simulink model "Ultrafiltration"  (R2025b)
settings: Solver=FixedStepAuto  StartTime=0.0  StopTime=1440  FixedStep=1  RelTol=1e-3
InitFcn:
  | initUF
  | tic;
StartFcn:
  | disp("Start...")
StopFcn:
  | disp("Stop...")
  | fprintf("SimTime: %.02f min", toc/60)
values from neighbouring files (symbols this model uses):
  BW_Max_Time = 90    [initUF.m]
  BW_Max_Vol_gal = 5000    [initUF.m]
  CEB_Max_Time = 1000    [initUF.m]
  CEB_Max_Vol_gal = 5000    [initUF.m]
  CIP_Max_Time = 15000    [initUF.m]
undefined symbols (not defined in the file or in its folder): LUT
libraries: simulink x30
(part 3 of 5)

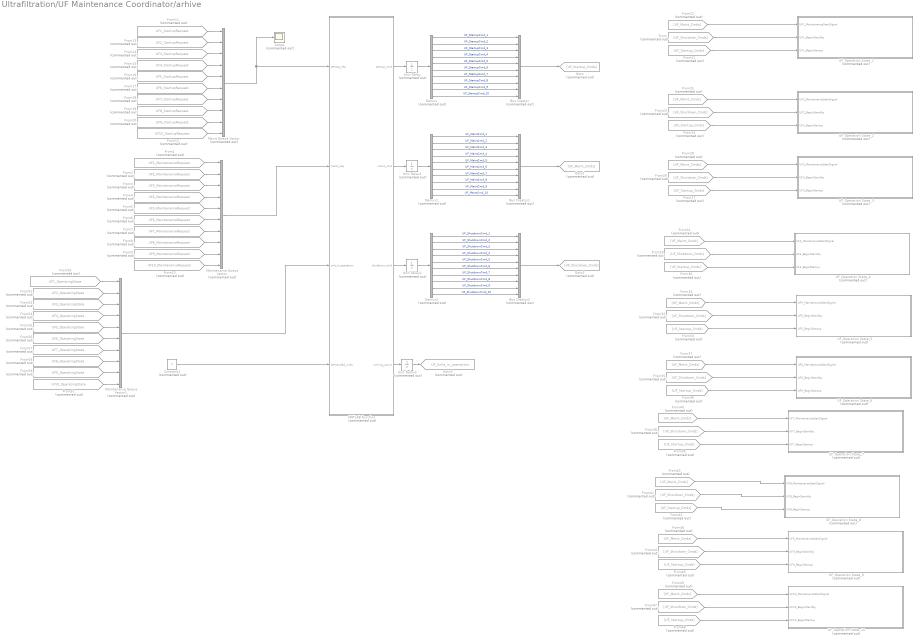
== system Ultrafiltration/UF Maintenance Coordinator/arhive ==
  Bus Creator : BusCreator  Commented=on  Inputs=10
  Bus Creator1 : BusCreator  Commented=on  Inputs=10
  Bus Creator2 : BusCreator  Commented=on  Inputs=10
  Constant1 : Constant  Commented=on  Value=7
  Demux : Demux  Commented=on  Outputs=10
  Demux1 : Demux  Commented=on  Outputs=10
  Demux2 : Demux  Commented=on  Outputs=10
  From{,23,26,29,32,35,38,41,44,47} (10 alike) : From  Commented=on  GotoTag=UF_Shutdown_Cmds
  From1 : From  Commented=on  GotoTag=UF1_MaintenanceRequest  TagVisibility=global
  From10 : From  Commented=on  GotoTag=UF10_MaintenanceRequest  TagVisibility=global
  From11 : From  Commented=on  GotoTag=UF1_StartupRequest  TagVisibility=global
  From12 : From  Commented=on  GotoTag=UF10_StartupRequest  TagVisibility=global
  From13 : From  Commented=on  GotoTag=UF2_StartupRequest  TagVisibility=global
  From14 : From  Commented=on  GotoTag=UF3_StartupRequest  TagVisibility=global
  From15 : From  Commented=on  GotoTag=UF4_StartupRequest  TagVisibility=global
  From16 : From  Commented=on  GotoTag=UF5_StartupRequest  TagVisibility=global
  From17 : From  Commented=on  GotoTag=UF6_StartupRequest  TagVisibility=global
  From18 : From  Commented=on  GotoTag=UF7_StartupRequest  TagVisibility=global
  From19 : From  Commented=on  GotoTag=UF8_StartupRequest  TagVisibility=global
  From2 : From  Commented=on  GotoTag=UF2_MaintenanceRequest  TagVisibility=global
  From20 : From  Commented=on  GotoTag=UF9_StartupRequest  TagVisibility=global
  From{21,24,27,30,33,36,39,42,45,48} (10 alike) : From  Commented=on  GotoTag=UF_Startup_Cmds
  From{22,25,28,31,34,37,40,43,46,49} (10 alike) : From  Commented=on  GotoTag=UF_Maint_Cmds
  From3 : From  Commented=on  GotoTag=UF3_MaintenanceRequest  TagVisibility=global
  From4 : From  Commented=on  GotoTag=UF4_MaintenanceRequest  TagVisibility=global
  From5 : From  Commented=on  GotoTag=UF5_MaintenanceRequest  TagVisibility=global
  From50 : From  Commented=on  GotoTag=UF1_OperatingState  TagVisibility=global
  From51 : From  Commented=on  GotoTag=UF10_OperatingState  TagVisibility=global
  From52 : From  Commented=on  GotoTag=UF2_OperatingState  TagVisibility=global
  From53 : From  Commented=on  GotoTag=UF3_OperatingState  TagVisibility=global
  From54 : From  Commented=on  GotoTag=UF4_OperatingState  TagVisibility=global
  From55 : From  Commented=on  GotoTag=UF5_OperatingState  TagVisibility=global
  From56 : From  Commented=on  GotoTag=UF6_OperatingState  TagVisibility=global
  From57 : From  Commented=on  GotoTag=UF7_OperatingState  TagVisibility=global
  From58 : From  Commented=on  GotoTag=UF8_OperatingState  TagVisibility=global
  From59 : From  Commented=on  GotoTag=UF9_OperatingState  TagVisibility=global
  From6 : From  Commented=on  GotoTag=UF6_MaintenanceRequest  TagVisibility=global
  From7 : From  Commented=on  GotoTag=UF7_MaintenanceRequest  TagVisibility=global
  From8 : From  Commented=on  GotoTag=UF8_MaintenanceRequest  TagVisibility=global
  From9 : From  Commented=on  GotoTag=UF9_MaintenanceRequest  TagVisibility=global
  Goto : Goto  Commented=on  GotoTag=UF_Startup_Cmds
  Goto1 : Goto  Commented=on  GotoTag=UF_Maint_Cmds
  Goto2 : Goto  Commented=on  GotoTag=UF_Shutdown_Cmds
  Goto3 : Goto  Commented=on  GotoTag=UF_Units_in_operations  TagVisibility=global
  MATLAB Function : MATLAB Function  Priority=100  Commented=on  TreatAsAtomicUnit=on
  Maint Queue Vector : Mux  Commented=on  Inputs=10
  Maintenance Queue Vector : Mux  Commented=on  Inputs=10
  Maintenance Queue Vector1 : Mux  Commented=on  Inputs=10
  Scope : Scope  Commented=on
      settings: ActiveDisplayYMinimum=0.31827009128781919  ActiveDisplayYMaximum=0.91954146390153213
  UF_Operation State_1 : Subsystem  Commented=on
  UF_Operation State_10 : Subsystem  Commented=on
  UF_Operation State_2 : Subsystem  Commented=on
  UF_Operation State_3 : Subsystem  Commented=on
  UF_Operation State_4 : Subsystem  Commented=on
  UF_Operation State_5 : Subsystem  Commented=on
  UF_Operation State_6 : Subsystem  Commented=on
  UF_Operation State_7 : Subsystem  Commented=on
  UF_Operation State_8 : Subsystem  Commented=on
  UF_Operation State_9 : Subsystem  Commented=on
  Unit Delay{,1..3} (4 alike) : UnitDelay  Commented=on  SampleTime=-1  HasFrameUpgradeWarning=on
  wires:
  Demux2/9 -> Bus Creator2/9  "UF_ShutdownCmd_9"
  From13/1 -> Maint Queue Vector/2
  From42/1 -> UF_Operation State_8/3(UF8_BeginStartup)
  From48/1 -> UF_Operation State_10/3(UF10_BeginStartup)
  Demux2/10 -> Bus Creator2/10  "UF_ShutdownCmd_10"
  From47/1 -> UF_Operation State_10/2(UF10_BeginStandby)
  Demux2/6 -> Bus Creator2/6  "UF_ShutdownCmd_6"
  Demux1/6 -> Bus Creator1/6  "UF_MaintCmd_6"
  From24/1 -> UF_Operation State_2/3(UF2_BeginStartup)
  Maintenance Queue Vector/1 -> MATLAB Function/2(maint_req)
  From1/1 -> Maintenance Queue Vector/1
  From23/1 -> UF_Operation State_2/2(UF2_BeginStandby)
  MATLAB Function/3(shutdown_cmd) -> Unit Delay2/1
  From30/1 -> UF_Operation State_4/3(UF4_BeginStartup)
  From57/1 -> Maintenance Queue Vector1/7
  Unit Delay/1 -> Demux/1
  Demux/10 -> Bus Creator/10  "UF_StartupCmd_10"
  From54/1 -> Maintenance Queue Vector1/4
  From45/1 -> UF_Operation State_9/3(UF9_BeginStartup)
  Demux1/2 -> Bus Creator1/2  "UF_MaintCmd_2"
  From7/1 -> Maintenance Queue Vector/7
  From58/1 -> Maintenance Queue Vector1/8
  From49/1 -> UF_Operation State_10/1(UF10_MaintenanceStartSignal)
  From29/1 -> UF_Operation State_4/2(UF4_BeginStandby)
  From6/1 -> Maintenance Queue Vector/6
  From10/1 -> Maintenance Queue Vector/10
  From56/1 -> Maintenance Queue Vector1/6
  From33/1 -> UF_Operation State_5/3(UF5_BeginStartup)
  From31/1 -> UF_Operation State_4/1(UF4_MaintenanceStartSignal)
  From/1 -> UF_Operation State_1/2(UF1_BeginStandby)
  From53/1 -> Maintenance Queue Vector1/3
  From34/1 -> UF_Operation State_5/1(UF5_MaintenanceStartSignal)
  Demux2/5 -> Bus Creator2/5  "UF_ShutdownCmd_5"
  Unit Delay3/1 -> Goto3/1
  From59/1 -> Maintenance Queue Vector1/9
  Demux/7 -> Bus Creator/7  "UF_StartupCmd_7"
  Maintenance Queue Vector1/1 -> MATLAB Function/3(unit_in_operation)
  Demux2/7 -> Bus Creator2/7  "UF_ShutdownCmd_7"
  From3/1 -> Maintenance Queue Vector/3
  From38/1 -> UF_Operation State_7/2(UF7_BeginStandby)
  From40/1 -> UF_Operation State_7/1(UF7_MaintenanceStartSignal)
  From26/1 -> UF_Operation State_3/2(UF3_BeginStandby)
  Bus Creator1/1 -> Goto1/1
  From2/1 -> Maintenance Queue Vector/2
  Demux2/3 -> Bus Creator2/3  "UF_ShutdownCmd_3"
  From39/1 -> UF_Operation State_7/3(UF7_BeginStartup)
  Demux1/9 -> Bus Creator1/9  "UF_MaintCmd_9"
  Demux2/2 -> Bus Creator2/2  "UF_ShutdownCmd_2"
  From46/1 -> UF_Operation State_9/1(UF9_MaintenanceStartSignal)
  From20/1 -> Maint Queue Vector/9
  Demux/4 -> Bus Creator/4  "UF_StartupCmd_4"
  Demux2/4 -> Bus Creator2/4  "UF_ShutdownCmd_4"
  Demux/5 -> Bus Creator/5  "UF_StartupCmd_5"
  Demux2/1 -> Bus Creator2/1  "UF_ShutdownCmd_1"
  From9/1 -> Maintenance Queue Vector/9
  From32/1 -> UF_Operation State_5/2(UF5_BeginStandby)
  Demux1/3 -> Bus Creator1/3  "UF_MaintCmd_3"
  Demux1/5 -> Bus Creator1/5  "UF_MaintCmd_5"
  From55/1 -> Maintenance Queue Vector1/5
  From4/1 -> Maintenance Queue Vector/4
  MATLAB Function/4(running_count) -> Unit Delay3/1
  Demux/6 -> Bus Creator/6  "UF_StartupCmd_6"
  From22/1 -> UF_Operation State_1/1(UF1_MaintenanceStartSignal)
  Demux/8 -> Bus Creator/8  "UF_StartupCmd_8"
  Demux/9 -> Bus Creator/9  "UF_StartupCmd_9"
  From8/1 -> Maintenance Queue Vector/8
  Demux1/1 -> Bus Creator1/1  "UF_MaintCmd_1"
  Demux1/10 -> Bus Creator1/10  "UF_MaintCmd_10"
  From50/1 -> Maintenance Queue Vector1/1
  Demux1/4 -> Bus Creator1/4  "UF_MaintCmd_4"
  MATLAB Function/1(startup_cmd) -> Unit Delay/1
  From52/1 -> Maintenance Queue Vector1/2
  From27/1 -> UF_Operation State_3/3(UF3_BeginStartup)
  From15/1 -> Maint Queue Vector/4
  From51/1 -> Maintenance Queue Vector1/10
  From36/1 -> UF_Operation State_6/3(UF6_BeginStartup)
  MATLAB Function/2(maint_cmd) -> Unit Delay1/1
  Unit Delay2/1 -> Demux2/1
  From43/1 -> UF_Operation State_8/1(UF8_MaintenanceStartSignal)
  From28/1 -> UF_Operation State_3/1(UF3_MaintenanceStartSignal)
  Demux2/8 -> Bus Creator2/8  "UF_ShutdownCmd_8"
  Demux/2 -> Bus Creator/2  "UF_StartupCmd_2"
  From35/1 -> UF_Operation State_6/2(UF6_BeginStandby)
  Bus Creator2/1 -> Goto2/1
  Bus Creator/1 -> Goto/1
  From37/1 -> UF_Operation State_6/1(UF6_MaintenanceStartSignal)
  Constant1/1 -> MATLAB Function/4(demanded_units)
  Demux1/8 -> Bus Creator1/8  "UF_MaintCmd_8"
  From25/1 -> UF_Operation State_2/1(UF2_MaintenanceStartSignal)
  From44/1 -> UF_Operation State_9/2(UF9_BeginStandby)
  Demux1/7 -> Bus Creator1/7  "UF_MaintCmd_7"
  Demux/3 -> Bus Creator/3  "UF_StartupCmd_3"
  Demux/1 -> Bus Creator/1  "UF_StartupCmd_1"
  From41/1 -> UF_Operation State_8/2(UF8_BeginStandby)
  From21/1 -> UF_Operation State_1/3(UF1_BeginStartup)
  From5/1 -> Maintenance Queue Vector/5
  Unit Delay1/1 -> Demux1/1
  From16/1 -> Maint Queue Vector/5
  From17/1 -> Maint Queue Vector/6
  From19/1 -> Maint Queue Vector/8
  From11/1 -> Maint Queue Vector/1
  From12/1 -> Maint Queue Vector/10
  From18/1 -> Maint Queue Vector/7
  Maint Queue Vector/1 -> Scope/1, MATLAB Function/1(startup_req)
  From14/1 -> Maint Queue Vector/3

== system Ultrafiltration/UF1/Subsystem ==
  note: The GAM utilizes smoothing functions to generate non-interacting linear regressions between the parameters. The format of the equation is as such:
      | $y = \beta_0 + \sum_{n=1}^N{f_n(x_n)}\\ f_n(x_n) = \beta_{n}*sm_n(x_n)$
      | where f_n is the weighted smoothing function for variable n across the set N. Each 1-D lookup table below represents the weighted smooth function output for the respective variable. This GAM lookup table approach provided a more computationally efficient method to predict using the GAM at very minor losses in fidelity ( ~0.1% MAPE from raw GAM outputs across a test set).
  t_BW : Inport
  t_CEB : Inport  Port=2
  t_CIP : Inport  Port=3
  V_BW : Inport  Port=4
  V_CEB : Inport  Port=5
  Feed Turbidity : Inport  Port=6
  T : Inport  Port=7
  B1: t_BW : Lookup_n-D  NumberOfTableDimensions=1  BreakpointsForDimension1=LUT.breakpoints(:,3)  Table=LUT.values(:,3)  ExtrapMethod=Clip  InternalRulePriority=Speed  RndMeth=Simplest
  B2: t_CEB : Lookup_n-D  NumberOfTableDimensions=1  BreakpointsForDimension1=LUT.breakpoints(:,5)  Table=LUT.values(:,5)  ExtrapMethod=Clip  InternalRulePriority=Speed  RndMeth=Simplest
  B3: t_CIP : Lookup_n-D  NumberOfTableDimensions=1  BreakpointsForDimension1=LUT.breakpoints(:,4)  Table=LUT.values(:,4)  ExtrapMethod=Clip  InternalRulePriority=Speed  RndMeth=Simplest
  B4: V_BW : Lookup_n-D  NumberOfTableDimensions=1  BreakpointsForDimension1=LUT.breakpoints(:,6)  Table=LUT.values(:,6)  ExtrapMethod=Clip  InternalRulePriority=Speed  RndMeth=Simplest
  B5: V_CEB : Lookup_n-D  NumberOfTableDimensions=1  BreakpointsForDimension1=LUT.breakpoints(:,7)  Table=LUT.values(:,7)  ExtrapMethod=Clip  InternalRulePriority=Speed  RndMeth=Simplest
  B6: Turbidity : Lookup_n-D  NumberOfTableDimensions=1  BreakpointsForDimension1=LUT.breakpoints(:,1)  Table=LUT.values(:,1)  ExtrapMethod=Clip  InternalRulePriority=Speed  RndMeth=Simplest
  B7: Temperature : Lookup_n-D  NumberOfTableDimensions=1  BreakpointsForDimension1=LUT.breakpoints(:,2)  Table=LUT.values(:,2)  ExtrapMethod=Clip  InternalRulePriority=Speed  RndMeth=Simplest
  Intercept : Constant  Value=LUT.intercept
  Sum : Sum  Inputs=++++++++
  A_UF : Outport
  wires:
  Sum/1 -> A_UF/1
  t_BW/1 -> B1: t_BW/1
  B1: t_BW/1 -> Sum/2
  Intercept/1 -> Sum/1
  t_CEB/1 -> B2: t_CEB/1
  B2: t_CEB/1 -> Sum/3
  t_CIP/1 -> B3: t_CIP/1
  B3: t_CIP/1 -> Sum/4
  V_BW/1 -> B4: V_BW/1
  B4: V_BW/1 -> Sum/5
  V_CEB/1 -> B5: V_CEB/1
  B5: V_CEB/1 -> Sum/6
  B6: Turbidity/1 -> Sum/7
  Feed Turbidity/1 -> B6: Turbidity/1
  T/1 -> B7: Temperature/1
  B7: Temperature/1 -> Sum/8

== system Ultrafiltration/UF10/Subsystem ==
  note: The GAM utilizes smoothing functions to generate non-interacting linear regressions between the parameters. The format of the equation is as such:
      | $y = \beta_0 + \sum_{n=1}^N{f_n(x_n)}\\ f_n(x_n) = \beta_{n}*sm_n(x_n)$
      | where f_n is the weighted smoothing function for variable n across the set N. Each 1-D lookup table below represents the weighted smooth function output for the respective variable. This GAM lookup table approach provided a more computationally efficient method to predict using the GAM at very minor losses in fidelity ( ~0.1% MAPE from raw GAM outputs across a test set).
  t_BW : Inport
  t_CEB : Inport  Port=2
  t_CIP : Inport  Port=3
  V_BW : Inport  Port=4
  V_CEB : Inport  Port=5
  Feed Turbidity : Inport  Port=6
  T : Inport  Port=7
  B1: t_BW : Lookup_n-D  NumberOfTableDimensions=1  BreakpointsForDimension1=LUT.breakpoints(:,3)  Table=LUT.values(:,3)  ExtrapMethod=Clip  InternalRulePriority=Speed  RndMeth=Simplest
  B2: t_CEB : Lookup_n-D  NumberOfTableDimensions=1  BreakpointsForDimension1=LUT.breakpoints(:,5)  Table=LUT.values(:,5)  ExtrapMethod=Clip  InternalRulePriority=Speed  RndMeth=Simplest
  B3: t_CIP : Lookup_n-D  NumberOfTableDimensions=1  BreakpointsForDimension1=LUT.breakpoints(:,4)  Table=LUT.values(:,4)  ExtrapMethod=Clip  InternalRulePriority=Speed  RndMeth=Simplest
  B4: V_BW : Lookup_n-D  NumberOfTableDimensions=1  BreakpointsForDimension1=LUT.breakpoints(:,6)  Table=LUT.values(:,6)  ExtrapMethod=Clip  InternalRulePriority=Speed  RndMeth=Simplest
  B5: V_CEB : Lookup_n-D  NumberOfTableDimensions=1  BreakpointsForDimension1=LUT.breakpoints(:,7)  Table=LUT.values(:,7)  ExtrapMethod=Clip  InternalRulePriority=Speed  RndMeth=Simplest
  B6: Turbidity : Lookup_n-D  NumberOfTableDimensions=1  BreakpointsForDimension1=LUT.breakpoints(:,1)  Table=LUT.values(:,1)  ExtrapMethod=Clip  InternalRulePriority=Speed  RndMeth=Simplest
  B7: Temperature : Lookup_n-D  NumberOfTableDimensions=1  BreakpointsForDimension1=LUT.breakpoints(:,2)  Table=LUT.values(:,2)  ExtrapMethod=Clip  InternalRulePriority=Speed  RndMeth=Simplest
  Intercept : Constant  Value=LUT.intercept
  Sum : Sum  Inputs=++++++++
  A_UF : Outport
  wires:
  Sum/1 -> A_UF/1
  t_BW/1 -> B1: t_BW/1
  B1: t_BW/1 -> Sum/2
  Intercept/1 -> Sum/1
  t_CEB/1 -> B2: t_CEB/1
  B2: t_CEB/1 -> Sum/3
  t_CIP/1 -> B3: t_CIP/1
  B3: t_CIP/1 -> Sum/4
  V_BW/1 -> B4: V_BW/1
  B4: V_BW/1 -> Sum/5
  V_CEB/1 -> B5: V_CEB/1
  B5: V_CEB/1 -> Sum/6
  B6: Turbidity/1 -> Sum/7
  Feed Turbidity/1 -> B6: Turbidity/1
  T/1 -> B7: Temperature/1
  B7: Temperature/1 -> Sum/8

== system Ultrafiltration/UF2/Subsystem ==
  note: The GAM utilizes smoothing functions to generate non-interacting linear regressions between the parameters. The format of the equation is as such:
      | $y = \beta_0 + \sum_{n=1}^N{f_n(x_n)}\\ f_n(x_n) = \beta_{n}*sm_n(x_n)$
      | where f_n is the weighted smoothing function for variable n across the set N. Each 1-D lookup table below represents the weighted smooth function output for the respective variable. This GAM lookup table approach provided a more computationally efficient method to predict using the GAM at very minor losses in fidelity ( ~0.1% MAPE from raw GAM outputs across a test set).
  t_BW : Inport
  t_CEB : Inport  Port=2
  t_CIP : Inport  Port=3
  V_BW : Inport  Port=4
  V_CEB : Inport  Port=5
  Feed Turbidity : Inport  Port=6
  T : Inport  Port=7
  B1: t_BW : Lookup_n-D  NumberOfTableDimensions=1  BreakpointsForDimension1=LUT.breakpoints(:,3)  Table=LUT.values(:,3)  ExtrapMethod=Clip  InternalRulePriority=Speed  RndMeth=Simplest
  B2: t_CEB : Lookup_n-D  NumberOfTableDimensions=1  BreakpointsForDimension1=LUT.breakpoints(:,5)  Table=LUT.values(:,5)  ExtrapMethod=Clip  InternalRulePriority=Speed  RndMeth=Simplest
  B3: t_CIP : Lookup_n-D  NumberOfTableDimensions=1  BreakpointsForDimension1=LUT.breakpoints(:,4)  Table=LUT.values(:,4)  ExtrapMethod=Clip  InternalRulePriority=Speed  RndMeth=Simplest
  B4: V_BW : Lookup_n-D  NumberOfTableDimensions=1  BreakpointsForDimension1=LUT.breakpoints(:,6)  Table=LUT.values(:,6)  ExtrapMethod=Clip  InternalRulePriority=Speed  RndMeth=Simplest
  B5: V_CEB : Lookup_n-D  NumberOfTableDimensions=1  BreakpointsForDimension1=LUT.breakpoints(:,7)  Table=LUT.values(:,7)  ExtrapMethod=Clip  InternalRulePriority=Speed  RndMeth=Simplest
  B6: Turbidity : Lookup_n-D  NumberOfTableDimensions=1  BreakpointsForDimension1=LUT.breakpoints(:,1)  Table=LUT.values(:,1)  ExtrapMethod=Clip  InternalRulePriority=Speed  RndMeth=Simplest
  B7: Temperature : Lookup_n-D  NumberOfTableDimensions=1  BreakpointsForDimension1=LUT.breakpoints(:,2)  Table=LUT.values(:,2)  ExtrapMethod=Clip  InternalRulePriority=Speed  RndMeth=Simplest
  Intercept : Constant  Value=LUT.intercept
  Sum : Sum  Inputs=++++++++
  A_UF : Outport
  wires:
  Sum/1 -> A_UF/1
  t_BW/1 -> B1: t_BW/1
  B1: t_BW/1 -> Sum/2
  Intercept/1 -> Sum/1
  t_CEB/1 -> B2: t_CEB/1
  B2: t_CEB/1 -> Sum/3
  t_CIP/1 -> B3: t_CIP/1
  B3: t_CIP/1 -> Sum/4
  V_BW/1 -> B4: V_BW/1
  B4: V_BW/1 -> Sum/5
  V_CEB/1 -> B5: V_CEB/1
  B5: V_CEB/1 -> Sum/6
  B6: Turbidity/1 -> Sum/7
  Feed Turbidity/1 -> B6: Turbidity/1
  T/1 -> B7: Temperature/1
  B7: Temperature/1 -> Sum/8

== system Ultrafiltration/UF3/Subsystem ==
  note: The GAM utilizes smoothing functions to generate non-interacting linear regressions between the parameters. The format of the equation is as such:
      | $y = \beta_0 + \sum_{n=1}^N{f_n(x_n)}\\ f_n(x_n) = \beta_{n}*sm_n(x_n)$
      | where f_n is the weighted smoothing function for variable n across the set N. Each 1-D lookup table below represents the weighted smooth function output for the respective variable. This GAM lookup table approach provided a more computationally efficient method to predict using the GAM at very minor losses in fidelity ( ~0.1% MAPE from raw GAM outputs across a test set).
  t_BW : Inport
  t_CEB : Inport  Port=2
  t_CIP : Inport  Port=3
  V_BW : Inport  Port=4
  V_CEB : Inport  Port=5
  Feed Turbidity : Inport  Port=6
  T : Inport  Port=7
  B1: t_BW : Lookup_n-D  NumberOfTableDimensions=1  BreakpointsForDimension1=LUT.breakpoints(:,3)  Table=LUT.values(:,3)  ExtrapMethod=Clip  InternalRulePriority=Speed  RndMeth=Simplest
  B2: t_CEB : Lookup_n-D  NumberOfTableDimensions=1  BreakpointsForDimension1=LUT.breakpoints(:,5)  Table=LUT.values(:,5)  ExtrapMethod=Clip  InternalRulePriority=Speed  RndMeth=Simplest
  B3: t_CIP : Lookup_n-D  NumberOfTableDimensions=1  BreakpointsForDimension1=LUT.breakpoints(:,4)  Table=LUT.values(:,4)  ExtrapMethod=Clip  InternalRulePriority=Speed  RndMeth=Simplest
  B4: V_BW : Lookup_n-D  NumberOfTableDimensions=1  BreakpointsForDimension1=LUT.breakpoints(:,6)  Table=LUT.values(:,6)  ExtrapMethod=Clip  InternalRulePriority=Speed  RndMeth=Simplest
  B5: V_CEB : Lookup_n-D  NumberOfTableDimensions=1  BreakpointsForDimension1=LUT.breakpoints(:,7)  Table=LUT.values(:,7)  ExtrapMethod=Clip  InternalRulePriority=Speed  RndMeth=Simplest
  B6: Turbidity : Lookup_n-D  NumberOfTableDimensions=1  BreakpointsForDimension1=LUT.breakpoints(:,1)  Table=LUT.values(:,1)  ExtrapMethod=Clip  InternalRulePriority=Speed  RndMeth=Simplest
  B7: Temperature : Lookup_n-D  NumberOfTableDimensions=1  BreakpointsForDimension1=LUT.breakpoints(:,2)  Table=LUT.values(:,2)  ExtrapMethod=Clip  InternalRulePriority=Speed  RndMeth=Simplest
  Intercept : Constant  Value=LUT.intercept
  Sum : Sum  Inputs=++++++++
  A_UF : Outport
  wires:
  Sum/1 -> A_UF/1
  t_BW/1 -> B1: t_BW/1
  B1: t_BW/1 -> Sum/2
  Intercept/1 -> Sum/1
  t_CEB/1 -> B2: t_CEB/1
  B2: t_CEB/1 -> Sum/3
  t_CIP/1 -> B3: t_CIP/1
  B3: t_CIP/1 -> Sum/4
  V_BW/1 -> B4: V_BW/1
  B4: V_BW/1 -> Sum/5
  V_CEB/1 -> B5: V_CEB/1
  B5: V_CEB/1 -> Sum/6
  B6: Turbidity/1 -> Sum/7
  Feed Turbidity/1 -> B6: Turbidity/1
  T/1 -> B7: Temperature/1
  B7: Temperature/1 -> Sum/8

== system Ultrafiltration/UF4/Subsystem ==
  note: The GAM utilizes smoothing functions to generate non-interacting linear regressions between the parameters. The format of the equation is as such:
      | $y = \beta_0 + \sum_{n=1}^N{f_n(x_n)}\\ f_n(x_n) = \beta_{n}*sm_n(x_n)$
      | where f_n is the weighted smoothing function for variable n across the set N. Each 1-D lookup table below represents the weighted smooth function output for the respective variable. This GAM lookup table approach provided a more computationally efficient method to predict using the GAM at very minor losses in fidelity ( ~0.1% MAPE from raw GAM outputs across a test set).
  t_BW : Inport
  t_CEB : Inport  Port=2
  t_CIP : Inport  Port=3
  V_BW : Inport  Port=4
  V_CEB : Inport  Port=5
  Feed Turbidity : Inport  Port=6
  T : Inport  Port=7
  B1: t_BW : Lookup_n-D  NumberOfTableDimensions=1  BreakpointsForDimension1=LUT.breakpoints(:,3)  Table=LUT.values(:,3)  ExtrapMethod=Clip  InternalRulePriority=Speed  RndMeth=Simplest
  B2: t_CEB : Lookup_n-D  NumberOfTableDimensions=1  BreakpointsForDimension1=LUT.breakpoints(:,5)  Table=LUT.values(:,5)  ExtrapMethod=Clip  InternalRulePriority=Speed  RndMeth=Simplest
  B3: t_CIP : Lookup_n-D  NumberOfTableDimensions=1  BreakpointsForDimension1=LUT.breakpoints(:,4)  Table=LUT.values(:,4)  ExtrapMethod=Clip  InternalRulePriority=Speed  RndMeth=Simplest
  B4: V_BW : Lookup_n-D  NumberOfTableDimensions=1  BreakpointsForDimension1=LUT.breakpoints(:,6)  Table=LUT.values(:,6)  ExtrapMethod=Clip  InternalRulePriority=Speed  RndMeth=Simplest
  B5: V_CEB : Lookup_n-D  NumberOfTableDimensions=1  BreakpointsForDimension1=LUT.breakpoints(:,7)  Table=LUT.values(:,7)  ExtrapMethod=Clip  InternalRulePriority=Speed  RndMeth=Simplest
  B6: Turbidity : Lookup_n-D  NumberOfTableDimensions=1  BreakpointsForDimension1=LUT.breakpoints(:,1)  Table=LUT.values(:,1)  ExtrapMethod=Clip  InternalRulePriority=Speed  RndMeth=Simplest
  B7: Temperature : Lookup_n-D  NumberOfTableDimensions=1  BreakpointsForDimension1=LUT.breakpoints(:,2)  Table=LUT.values(:,2)  ExtrapMethod=Clip  InternalRulePriority=Speed  RndMeth=Simplest
  Intercept : Constant  Value=LUT.intercept
  Sum : Sum  Inputs=++++++++
  A_UF : Outport
  wires:
  Sum/1 -> A_UF/1
  t_BW/1 -> B1: t_BW/1
  B1: t_BW/1 -> Sum/2
  Intercept/1 -> Sum/1
  t_CEB/1 -> B2: t_CEB/1
  B2: t_CEB/1 -> Sum/3
  t_CIP/1 -> B3: t_CIP/1
  B3: t_CIP/1 -> Sum/4
  V_BW/1 -> B4: V_BW/1
  B4: V_BW/1 -> Sum/5
  V_CEB/1 -> B5: V_CEB/1
  B5: V_CEB/1 -> Sum/6
  B6: Turbidity/1 -> Sum/7
  Feed Turbidity/1 -> B6: Turbidity/1
  T/1 -> B7: Temperature/1
  B7: Temperature/1 -> Sum/8

== system Ultrafiltration/UF5/Subsystem ==
  note: The GAM utilizes smoothing functions to generate non-interacting linear regressions between the parameters. The format of the equation is as such:
      | $y = \beta_0 + \sum_{n=1}^N{f_n(x_n)}\\ f_n(x_n) = \beta_{n}*sm_n(x_n)$
      | where f_n is the weighted smoothing function for variable n across the set N. Each 1-D lookup table below represents the weighted smooth function output for the respective variable. This GAM lookup table approach provided a more computationally efficient method to predict using the GAM at very minor losses in fidelity ( ~0.1% MAPE from raw GAM outputs across a test set).
  t_BW : Inport
  t_CEB : Inport  Port=2
  t_CIP : Inport  Port=3
  V_BW : Inport  Port=4
  V_CEB : Inport  Port=5
  Feed Turbidity : Inport  Port=6
  T : Inport  Port=7
  B1: t_BW : Lookup_n-D  NumberOfTableDimensions=1  BreakpointsForDimension1=LUT.breakpoints(:,3)  Table=LUT.values(:,3)  ExtrapMethod=Clip  InternalRulePriority=Speed  RndMeth=Simplest
  B2: t_CEB : Lookup_n-D  NumberOfTableDimensions=1  BreakpointsForDimension1=LUT.breakpoints(:,5)  Table=LUT.values(:,5)  ExtrapMethod=Clip  InternalRulePriority=Speed  RndMeth=Simplest
  B3: t_CIP : Lookup_n-D  NumberOfTableDimensions=1  BreakpointsForDimension1=LUT.breakpoints(:,4)  Table=LUT.values(:,4)  ExtrapMethod=Clip  InternalRulePriority=Speed  RndMeth=Simplest
  B4: V_BW : Lookup_n-D  NumberOfTableDimensions=1  BreakpointsForDimension1=LUT.breakpoints(:,6)  Table=LUT.values(:,6)  ExtrapMethod=Clip  InternalRulePriority=Speed  RndMeth=Simplest
  B5: V_CEB : Lookup_n-D  NumberOfTableDimensions=1  BreakpointsForDimension1=LUT.breakpoints(:,7)  Table=LUT.values(:,7)  ExtrapMethod=Clip  InternalRulePriority=Speed  RndMeth=Simplest
  B6: Turbidity : Lookup_n-D  NumberOfTableDimensions=1  BreakpointsForDimension1=LUT.breakpoints(:,1)  Table=LUT.values(:,1)  ExtrapMethod=Clip  InternalRulePriority=Speed  RndMeth=Simplest
  B7: Temperature : Lookup_n-D  NumberOfTableDimensions=1  BreakpointsForDimension1=LUT.breakpoints(:,2)  Table=LUT.values(:,2)  ExtrapMethod=Clip  InternalRulePriority=Speed  RndMeth=Simplest
  Intercept : Constant  Value=LUT.intercept
  Sum : Sum  Inputs=++++++++
  A_UF : Outport
  wires:
  Sum/1 -> A_UF/1
  t_BW/1 -> B1: t_BW/1
  B1: t_BW/1 -> Sum/2
  Intercept/1 -> Sum/1
  t_CEB/1 -> B2: t_CEB/1
  B2: t_CEB/1 -> Sum/3
  t_CIP/1 -> B3: t_CIP/1
  B3: t_CIP/1 -> Sum/4
  V_BW/1 -> B4: V_BW/1
  B4: V_BW/1 -> Sum/5
  V_CEB/1 -> B5: V_CEB/1
  B5: V_CEB/1 -> Sum/6
  B6: Turbidity/1 -> Sum/7
  Feed Turbidity/1 -> B6: Turbidity/1
  T/1 -> B7: Temperature/1
  B7: Temperature/1 -> Sum/8

== system Ultrafiltration/UF6/Subsystem ==
  note: The GAM utilizes smoothing functions to generate non-interacting linear regressions between the parameters. The format of the equation is as such:
      | $y = \beta_0 + \sum_{n=1}^N{f_n(x_n)}\\ f_n(x_n) = \beta_{n}*sm_n(x_n)$
      | where f_n is the weighted smoothing function for variable n across the set N. Each 1-D lookup table below represents the weighted smooth function output for the respective variable. This GAM lookup table approach provided a more computationally efficient method to predict using the GAM at very minor losses in fidelity ( ~0.1% MAPE from raw GAM outputs across a test set).
  t_BW : Inport
  t_CEB : Inport  Port=2
  t_CIP : Inport  Port=3
  V_BW : Inport  Port=4
  V_CEB : Inport  Port=5
  Feed Turbidity : Inport  Port=6
  T : Inport  Port=7
  B1: t_BW : Lookup_n-D  NumberOfTableDimensions=1  BreakpointsForDimension1=LUT.breakpoints(:,3)  Table=LUT.values(:,3)  ExtrapMethod=Clip  InternalRulePriority=Speed  RndMeth=Simplest
  B2: t_CEB : Lookup_n-D  NumberOfTableDimensions=1  BreakpointsForDimension1=LUT.breakpoints(:,5)  Table=LUT.values(:,5)  ExtrapMethod=Clip  InternalRulePriority=Speed  RndMeth=Simplest
  B3: t_CIP : Lookup_n-D  NumberOfTableDimensions=1  BreakpointsForDimension1=LUT.breakpoints(:,4)  Table=LUT.values(:,4)  ExtrapMethod=Clip  InternalRulePriority=Speed  RndMeth=Simplest
  B4: V_BW : Lookup_n-D  NumberOfTableDimensions=1  BreakpointsForDimension1=LUT.breakpoints(:,6)  Table=LUT.values(:,6)  ExtrapMethod=Clip  InternalRulePriority=Speed  RndMeth=Simplest
  B5: V_CEB : Lookup_n-D  NumberOfTableDimensions=1  BreakpointsForDimension1=LUT.breakpoints(:,7)  Table=LUT.values(:,7)  ExtrapMethod=Clip  InternalRulePriority=Speed  RndMeth=Simplest
  B6: Turbidity : Lookup_n-D  NumberOfTableDimensions=1  BreakpointsForDimension1=LUT.breakpoints(:,1)  Table=LUT.values(:,1)  ExtrapMethod=Clip  InternalRulePriority=Speed  RndMeth=Simplest
  B7: Temperature : Lookup_n-D  NumberOfTableDimensions=1  BreakpointsForDimension1=LUT.breakpoints(:,2)  Table=LUT.values(:,2)  ExtrapMethod=Clip  InternalRulePriority=Speed  RndMeth=Simplest
  Intercept : Constant  Value=LUT.intercept
  Sum : Sum  Inputs=++++++++
  A_UF : Outport
  wires:
  Sum/1 -> A_UF/1
  t_BW/1 -> B1: t_BW/1
  B1: t_BW/1 -> Sum/2
  Intercept/1 -> Sum/1
  t_CEB/1 -> B2: t_CEB/1
  B2: t_CEB/1 -> Sum/3
  t_CIP/1 -> B3: t_CIP/1
  B3: t_CIP/1 -> Sum/4
  V_BW/1 -> B4: V_BW/1
  B4: V_BW/1 -> Sum/5
  V_CEB/1 -> B5: V_CEB/1
  B5: V_CEB/1 -> Sum/6
  B6: Turbidity/1 -> Sum/7
  Feed Turbidity/1 -> B6: Turbidity/1
  T/1 -> B7: Temperature/1
  B7: Temperature/1 -> Sum/8

== system Ultrafiltration/UF7/Subsystem ==
  note: The GAM utilizes smoothing functions to generate non-interacting linear regressions between the parameters. The format of the equation is as such:
      | $y = \beta_0 + \sum_{n=1}^N{f_n(x_n)}\\ f_n(x_n) = \beta_{n}*sm_n(x_n)$
      | where f_n is the weighted smoothing function for variable n across the set N. Each 1-D lookup table below represents the weighted smooth function output for the respective variable. This GAM lookup table approach provided a more computationally efficient method to predict using the GAM at very minor losses in fidelity ( ~0.1% MAPE from raw GAM outputs across a test set).
  t_BW : Inport
  t_CEB : Inport  Port=2
  t_CIP : Inport  Port=3
  V_BW : Inport  Port=4
  V_CEB : Inport  Port=5
  Feed Turbidity : Inport  Port=6
  T : Inport  Port=7
  B1: t_BW : Lookup_n-D  NumberOfTableDimensions=1  BreakpointsForDimension1=LUT.breakpoints(:,3)  Table=LUT.values(:,3)  ExtrapMethod=Clip  InternalRulePriority=Speed  RndMeth=Simplest
  B2: t_CEB : Lookup_n-D  NumberOfTableDimensions=1  BreakpointsForDimension1=LUT.breakpoints(:,5)  Table=LUT.values(:,5)  ExtrapMethod=Clip  InternalRulePriority=Speed  RndMeth=Simplest
  B3: t_CIP : Lookup_n-D  NumberOfTableDimensions=1  BreakpointsForDimension1=LUT.breakpoints(:,4)  Table=LUT.values(:,4)  ExtrapMethod=Clip  InternalRulePriority=Speed  RndMeth=Simplest
  B4: V_BW : Lookup_n-D  NumberOfTableDimensions=1  BreakpointsForDimension1=LUT.breakpoints(:,6)  Table=LUT.values(:,6)  ExtrapMethod=Clip  InternalRulePriority=Speed  RndMeth=Simplest
  B5: V_CEB : Lookup_n-D  NumberOfTableDimensions=1  BreakpointsForDimension1=LUT.breakpoints(:,7)  Table=LUT.values(:,7)  ExtrapMethod=Clip  InternalRulePriority=Speed  RndMeth=Simplest
  B6: Turbidity : Lookup_n-D  NumberOfTableDimensions=1  BreakpointsForDimension1=LUT.breakpoints(:,1)  Table=LUT.values(:,1)  ExtrapMethod=Clip  InternalRulePriority=Speed  RndMeth=Simplest
  B7: Temperature : Lookup_n-D  NumberOfTableDimensions=1  BreakpointsForDimension1=LUT.breakpoints(:,2)  Table=LUT.values(:,2)  ExtrapMethod=Clip  InternalRulePriority=Speed  RndMeth=Simplest
  Intercept : Constant  Value=LUT.intercept
  Sum : Sum  Inputs=++++++++
  A_UF : Outport
  wires:
  Sum/1 -> A_UF/1
  t_BW/1 -> B1: t_BW/1
  B1: t_BW/1 -> Sum/2
  Intercept/1 -> Sum/1
  t_CEB/1 -> B2: t_CEB/1
  B2: t_CEB/1 -> Sum/3
  t_CIP/1 -> B3: t_CIP/1
  B3: t_CIP/1 -> Sum/4
  V_BW/1 -> B4: V_BW/1
  B4: V_BW/1 -> Sum/5
  V_CEB/1 -> B5: V_CEB/1
  B5: V_CEB/1 -> Sum/6
  B6: Turbidity/1 -> Sum/7
  Feed Turbidity/1 -> B6: Turbidity/1
  T/1 -> B7: Temperature/1
  B7: Temperature/1 -> Sum/8

== system Ultrafiltration/UF8/Subsystem ==
  note: The GAM utilizes smoothing functions to generate non-interacting linear regressions between the parameters. The format of the equation is as such:
      | $y = \beta_0 + \sum_{n=1}^N{f_n(x_n)}\\ f_n(x_n) = \beta_{n}*sm_n(x_n)$
      | where f_n is the weighted smoothing function for variable n across the set N. Each 1-D lookup table below represents the weighted smooth function output for the respective variable. This GAM lookup table approach provided a more computationally efficient method to predict using the GAM at very minor losses in fidelity ( ~0.1% MAPE from raw GAM outputs across a test set).
  t_BW : Inport
  t_CEB : Inport  Port=2
  t_CIP : Inport  Port=3
  V_BW : Inport  Port=4
  V_CEB : Inport  Port=5
  Feed Turbidity : Inport  Port=6
  T : Inport  Port=7
  B1: t_BW : Lookup_n-D  NumberOfTableDimensions=1  BreakpointsForDimension1=LUT.breakpoints(:,3)  Table=LUT.values(:,3)  ExtrapMethod=Clip  InternalRulePriority=Speed  RndMeth=Simplest
  B2: t_CEB : Lookup_n-D  NumberOfTableDimensions=1  BreakpointsForDimension1=LUT.breakpoints(:,5)  Table=LUT.values(:,5)  ExtrapMethod=Clip  InternalRulePriority=Speed  RndMeth=Simplest
  B3: t_CIP : Lookup_n-D  NumberOfTableDimensions=1  BreakpointsForDimension1=LUT.breakpoints(:,4)  Table=LUT.values(:,4)  ExtrapMethod=Clip  InternalRulePriority=Speed  RndMeth=Simplest
  B4: V_BW : Lookup_n-D  NumberOfTableDimensions=1  BreakpointsForDimension1=LUT.breakpoints(:,6)  Table=LUT.values(:,6)  ExtrapMethod=Clip  InternalRulePriority=Speed  RndMeth=Simplest
  B5: V_CEB : Lookup_n-D  NumberOfTableDimensions=1  BreakpointsForDimension1=LUT.breakpoints(:,7)  Table=LUT.values(:,7)  ExtrapMethod=Clip  InternalRulePriority=Speed  RndMeth=Simplest
  B6: Turbidity : Lookup_n-D  NumberOfTableDimensions=1  BreakpointsForDimension1=LUT.breakpoints(:,1)  Table=LUT.values(:,1)  ExtrapMethod=Clip  InternalRulePriority=Speed  RndMeth=Simplest
  B7: Temperature : Lookup_n-D  NumberOfTableDimensions=1  BreakpointsForDimension1=LUT.breakpoints(:,2)  Table=LUT.values(:,2)  ExtrapMethod=Clip  InternalRulePriority=Speed  RndMeth=Simplest
  Intercept : Constant  Value=LUT.intercept
  Sum : Sum  Inputs=++++++++
  A_UF : Outport
  wires:
  Sum/1 -> A_UF/1
  t_BW/1 -> B1: t_BW/1
  B1: t_BW/1 -> Sum/2
  Intercept/1 -> Sum/1
  t_CEB/1 -> B2: t_CEB/1
  B2: t_CEB/1 -> Sum/3
  t_CIP/1 -> B3: t_CIP/1
  B3: t_CIP/1 -> Sum/4
  V_BW/1 -> B4: V_BW/1
  B4: V_BW/1 -> Sum/5
  V_CEB/1 -> B5: V_CEB/1
  B5: V_CEB/1 -> Sum/6
  B6: Turbidity/1 -> Sum/7
  Feed Turbidity/1 -> B6: Turbidity/1
  T/1 -> B7: Temperature/1
  B7: Temperature/1 -> Sum/8

== system Ultrafiltration/UF9/Subsystem ==
  note: The GAM utilizes smoothing functions to generate non-interacting linear regressions between the parameters. The format of the equation is as such:
      | $y = \beta_0 + \sum_{n=1}^N{f_n(x_n)}\\ f_n(x_n) = \beta_{n}*sm_n(x_n)$
      | where f_n is the weighted smoothing function for variable n across the set N. Each 1-D lookup table below represents the weighted smooth function output for the respective variable. This GAM lookup table approach provided a more computationally efficient method to predict using the GAM at very minor losses in fidelity ( ~0.1% MAPE from raw GAM outputs across a test set).
  t_BW : Inport
  t_CEB : Inport  Port=2
  t_CIP : Inport  Port=3
  V_BW : Inport  Port=4
  V_CEB : Inport  Port=5
  Feed Turbidity : Inport  Port=6
  T : Inport  Port=7
  B1: t_BW : Lookup_n-D  NumberOfTableDimensions=1  BreakpointsForDimension1=LUT.breakpoints(:,3)  Table=LUT.values(:,3)  ExtrapMethod=Clip  InternalRulePriority=Speed  RndMeth=Simplest
  B2: t_CEB : Lookup_n-D  NumberOfTableDimensions=1  BreakpointsForDimension1=LUT.breakpoints(:,5)  Table=LUT.values(:,5)  ExtrapMethod=Clip  InternalRulePriority=Speed  RndMeth=Simplest
  B3: t_CIP : Lookup_n-D  NumberOfTableDimensions=1  BreakpointsForDimension1=LUT.breakpoints(:,4)  Table=LUT.values(:,4)  ExtrapMethod=Clip  InternalRulePriority=Speed  RndMeth=Simplest
  B4: V_BW : Lookup_n-D  NumberOfTableDimensions=1  BreakpointsForDimension1=LUT.breakpoints(:,6)  Table=LUT.values(:,6)  ExtrapMethod=Clip  InternalRulePriority=Speed  RndMeth=Simplest
  B5: V_CEB : Lookup_n-D  NumberOfTableDimensions=1  BreakpointsForDimension1=LUT.breakpoints(:,7)  Table=LUT.values(:,7)  ExtrapMethod=Clip  InternalRulePriority=Speed  RndMeth=Simplest
  B6: Turbidity : Lookup_n-D  NumberOfTableDimensions=1  BreakpointsForDimension1=LUT.breakpoints(:,1)  Table=LUT.values(:,1)  ExtrapMethod=Clip  InternalRulePriority=Speed  RndMeth=Simplest
  B7: Temperature : Lookup_n-D  NumberOfTableDimensions=1  BreakpointsForDimension1=LUT.breakpoints(:,2)  Table=LUT.values(:,2)  ExtrapMethod=Clip  InternalRulePriority=Speed  RndMeth=Simplest
  Intercept : Constant  Value=LUT.intercept
  Sum : Sum  Inputs=++++++++
  A_UF : Outport
  wires:
  Sum/1 -> A_UF/1
  t_BW/1 -> B1: t_BW/1
  B1: t_BW/1 -> Sum/2
  Intercept/1 -> Sum/1
  t_CEB/1 -> B2: t_CEB/1
  B2: t_CEB/1 -> Sum/3
  t_CIP/1 -> B3: t_CIP/1
  B3: t_CIP/1 -> Sum/4
  V_BW/1 -> B4: V_BW/1
  B4: V_BW/1 -> Sum/5
  V_CEB/1 -> B5: V_CEB/1
  B5: V_CEB/1 -> Sum/6
  B6: Turbidity/1 -> Sum/7
  Feed Turbidity/1 -> B6: Turbidity/1
  T/1 -> B7: Temperature/1
  B7: Temperature/1 -> Sum/8

== system Ultrafiltration/UF Maintenance Coordinator/arhive/UF_Operation State_1 ==
  UF1_MaintenanceStartSignal : Inport
  UF1_BeginStandby : Inport  Port=2
  UF1_BeginStartup : Inport  Port=3
  Bus Creator : BusCreator  Inputs=2
  Bus Selector : BusSelector  OutputSignals=UF_ShutdownCmd_1
  Bus Selector1 : BusSelector  OutputSignals=UF_MaintCmd_1
  Bus Selector2 : BusSelector  OutputSignals=UF_StartupCmd_1
  Delay Reset Signal : Memory
  Delay Startup : Memory
  UF1_Maintenance State : Stateflow chart  TreatAsAtomicUnit=on
  tag scope: UF1_MaintenanceRequest=global, UF1_MaintenanceState=global, UF1_OperatingState=global, UF1_StartupRequest=global
  wires:
  UF1_Maintenance State/1(unit_in_maint_queue) -> [UF1_MaintenanceRequest]  "UF1_MaintenanceRequestQueue"
  Bus Creator/1 -> [UF1_MaintenanceState]
  Delay Startup/1 -> [UF1_OperatingState], Bus Creator/1  "UF1_OperationsState"
  UF1_Maintenance State/4(maintenance_completion_indicator) -> Delay Reset Signal/1  "UF1_MaintenanceCompletionSignal"
  [UF1_Maintenance_Request] -> UF1_Maintenance State/2(maint_req)
  Delay Reset Signal/1 -> Bus Creator/2  "UF1_MaintenanceCompletionSignal"
  UF1_Maintenance State/3(unit_in_operation) -> Delay Startup/1  "UF1_OperationsState"
  UF1_Maintenance State/2(unit_in_startup_queue) -> [UF1_StartupRequest]  "UF1_StartupRequestQueue"
  UF1_BeginStandby/1 -> Bus Selector/1  "UF1_BeginStandby"
  Bus Selector/1 -> UF1_Maintenance State/3(standby_cmd)  "<UF_ShutdownCmd_1>"
  UF1_MaintenanceStartSignal/1 -> Bus Selector1/1  "UF1_MaintenanceStartSignal"
  Bus Selector1/1 -> UF1_Maintenance State/1(maint_cmd)  "<UF_MaintCmd_1>"
  UF1_BeginStartup/1 -> Bus Selector2/1  "UF1_BeginStartup"
  Bus Selector2/1 -> UF1_Maintenance State/4(startup_cmd)  "<UF_StartupCmd_1>"

== system Ultrafiltration/UF Maintenance Coordinator/arhive/UF_Operation State_10 ==
  UF10_MaintenanceStartSignal : Inport
  UF10_BeginStandby : Inport  Port=2
  UF10_BeginStartup : Inport  Port=3
  Bus Creator : BusCreator  Inputs=2
  Bus Selector : BusSelector  OutputSignals=UF_ShutdownCmd_10
  Bus Selector10 : BusSelector  OutputSignals=UF_MaintCmd_10
  Bus Selector2 : BusSelector  OutputSignals=UF_StartupCmd_10
  Delay Reset Signal : Memory
  Delay Startup : Memory
  UF10_Maintenance State : Stateflow chart  TreatAsAtomicUnit=on
  tag scope: UF10_MaintenanceRequest=global, UF10_MaintenanceState=global, UF10_OperatingState=global, UF10_StartupRequest=global
  wires:
  UF10_Maintenance State/1(unit_in_maint_queue) -> [UF10_MaintenanceRequest]  "UF10_MaintenanceRequestQueue"
  Bus Creator/1 -> [UF10_MaintenanceState]
  Delay Startup/1 -> [UF10_OperatingState], Bus Creator/1  "UF10_OperationsState"
  UF10_Maintenance State/4(maintenance_completion_indicator) -> Delay Reset Signal/1  "UF10_MaintenanceCompletionSignal"
  [UF10_Maintenance_Request] -> UF10_Maintenance State/2(maint_req)
  Delay Reset Signal/1 -> Bus Creator/2  "UF10_MaintenanceCompletionSignal"
  UF10_Maintenance State/3(unit_in_operation) -> Delay Startup/1  "UF10_OperationsState"
  UF10_Maintenance State/2(unit_in_startup_queue) -> [UF10_StartupRequest]  "UF10_StartupRequestQueue"
  UF10_BeginStandby/1 -> Bus Selector/1  "UF10_BeginStandby"
  Bus Selector/1 -> UF10_Maintenance State/3(standby_cmd)  "<UF_ShutdownCmd_10>"
  UF10_MaintenanceStartSignal/1 -> Bus Selector10/1  "UF10_MaintenanceStartSignal"
  Bus Selector10/1 -> UF10_Maintenance State/1(maint_cmd)  "<UF_MaintCmd_10>"
  UF10_BeginStartup/1 -> Bus Selector2/1  "UF10_BeginStartup"
  Bus Selector2/1 -> UF10_Maintenance State/4(startup_cmd)  "<UF_StartupCmd_10>"

== system Ultrafiltration/UF Maintenance Coordinator/arhive/UF_Operation State_2 ==
  UF2_MaintenanceStartSignal : Inport
  UF2_BeginStandby : Inport  Port=2
  UF2_BeginStartup : Inport  Port=3
  Bus Creator : BusCreator  Inputs=2
  Bus Selector : BusSelector  OutputSignals=UF_ShutdownCmd_2
  Bus Selector1 : BusSelector  OutputSignals=UF_MaintCmd_2
  Bus Selector2 : BusSelector  OutputSignals=UF_StartupCmd_2
  Delay Reset Signal : Memory
  Delay Startup : Memory
  UF2_Maintenance State : Stateflow chart  TreatAsAtomicUnit=on
  tag scope: UF2_MaintenanceRequest=global, UF2_MaintenanceState=global, UF2_OperatingState=global, UF2_StartupRequest=global
  wires:
  UF2_Maintenance State/1(unit_in_maint_queue) -> [UF2_MaintenanceRequest]  "UF2_MaintenanceRequestQueue"
  Bus Creator/1 -> [UF2_MaintenanceState]
  UF2_Maintenance State/4(maintenance_completion_indicator) -> Delay Reset Signal/1  "UF2_MaintenanceCompletionSignal"
  [UF2_Maintenance_Request] -> UF2_Maintenance State/2(maint_req)
  Delay Reset Signal/1 -> Bus Creator/2  "UF2_MaintenanceCompletionSignal"
  UF2_Maintenance State/3(unit_in_operation) -> Delay Startup/1  "UF2_OperationsState"
  UF2_Maintenance State/2(unit_in_startup_queue) -> [UF2_StartupRequest]  "UF2_StartupRequestQueue"
  UF2_BeginStandby/1 -> Bus Selector/1  "UF2_BeginStandby"
  Bus Selector/1 -> UF2_Maintenance State/3(standby_cmd)  "<UF_ShutdownCmd_2>"
  UF2_MaintenanceStartSignal/1 -> Bus Selector1/1  "UF2_MaintenanceStartSignal"
  Bus Selector1/1 -> UF2_Maintenance State/1(maint_cmd)  "<UF_MaintCmd_2>"
  UF2_BeginStartup/1 -> Bus Selector2/1  "UF2_BeginStartup"
  Bus Selector2/1 -> UF2_Maintenance State/4(startup_cmd)  "<UF_StartupCmd_2>"
  Delay Startup/1 -> [UF2_OperatingState], Bus Creator/1  "UF2_OperationsState"

== system Ultrafiltration/UF Maintenance Coordinator/arhive/UF_Operation State_3 ==
  UF3_MaintenanceStartSignal : Inport
  UF3_BeginStandby : Inport  Port=2
  UF3_BeginStartup : Inport  Port=3
  Bus Creator : BusCreator  Inputs=2
  Bus Selector : BusSelector  OutputSignals=UF_ShutdownCmd_3
  Bus Selector2 : BusSelector  OutputSignals=UF_StartupCmd_3
  Bus Selector3 : BusSelector  OutputSignals=UF_MaintCmd_3
  Delay Reset Signal : Memory
  Delay Startup : Memory
  UF3_Maintenance State : Stateflow chart  TreatAsAtomicUnit=on
  tag scope: UF3_MaintenanceRequest=global, UF3_MaintenanceState=global, UF3_OperatingState=global, UF3_StartupRequest=global
  wires:
  UF3_Maintenance State/1(unit_in_maint_queue) -> [UF3_MaintenanceRequest]  "UF3_MaintenanceRequestQueue"
  Bus Creator/1 -> [UF3_MaintenanceState]
  Delay Startup/1 -> [UF3_OperatingState], Bus Creator/1  "UF3_OperationsState"
  UF3_Maintenance State/4(maintenance_completion_indicator) -> Delay Reset Signal/1  "UF3_MaintenanceCompletionSignal"
  [UF3_Maintenance_Request] -> UF3_Maintenance State/2(maint_req)
  Delay Reset Signal/1 -> Bus Creator/2  "UF3_MaintenanceCompletionSignal"
  UF3_Maintenance State/3(unit_in_operation) -> Delay Startup/1  "UF3_OperationsState"
  UF3_Maintenance State/2(unit_in_startup_queue) -> [UF3_StartupRequest]  "UF3_StartupRequestQueue"
  UF3_BeginStandby/1 -> Bus Selector/1  "UF3_BeginStandby"
  Bus Selector/1 -> UF3_Maintenance State/3(standby_cmd)  "<UF_ShutdownCmd_3>"
  UF3_MaintenanceStartSignal/1 -> Bus Selector3/1  "UF3_MaintenanceStartSignal"
  Bus Selector3/1 -> UF3_Maintenance State/1(maint_cmd)  "<UF_MaintCmd_3>"
  UF3_BeginStartup/1 -> Bus Selector2/1  "UF3_BeginStartup"
  Bus Selector2/1 -> UF3_Maintenance State/4(startup_cmd)  "<UF_StartupCmd_3>"

== system Ultrafiltration/UF Maintenance Coordinator/arhive/UF_Operation State_4 ==
  UF4_MaintenanceStartSignal : Inport
  UF4_BeginStandby : Inport  Port=2
  UF4_BeginStartup : Inport  Port=3
  Bus Creator : BusCreator  Inputs=2
  Bus Selector : BusSelector  OutputSignals=UF_ShutdownCmd_4
  Bus Selector2 : BusSelector  OutputSignals=UF_StartupCmd_4
  Bus Selector4 : BusSelector  OutputSignals=UF_MaintCmd_4
  Delay Reset Signal : Memory
  Delay Startup : Memory
  UF4_Maintenance State : Stateflow chart  TreatAsAtomicUnit=on
  tag scope: UF4_MaintenanceRequest=global, UF4_MaintenanceState=global, UF4_OperatingState=global, UF4_StartupRequest=global
  wires:
  UF4_Maintenance State/1(unit_in_maint_queue) -> [UF4_MaintenanceRequest]  "UF4_MaintenanceRequestQueue"
  Bus Creator/1 -> [UF4_MaintenanceState]
  Delay Startup/1 -> [UF4_OperatingState], Bus Creator/1  "UF4_OperationsState"
  UF4_Maintenance State/4(maintenance_completion_indicator) -> Delay Reset Signal/1  "UF4_MaintenanceCompletionSignal"
  [UF4_Maintenance_Request] -> UF4_Maintenance State/2(maint_req)
  Delay Reset Signal/1 -> Bus Creator/2  "UF4_MaintenanceCompletionSignal"
  UF4_Maintenance State/3(unit_in_operation) -> Delay Startup/1  "UF4_OperationsState"
  UF4_Maintenance State/2(unit_in_startup_queue) -> [UF4_StartupRequest]  "UF4_StartupRequestQueue"
  UF4_BeginStandby/1 -> Bus Selector/1  "UF4_BeginStandby"
  Bus Selector/1 -> UF4_Maintenance State/3(standby_cmd)  "<UF_ShutdownCmd_4>"
  UF4_MaintenanceStartSignal/1 -> Bus Selector4/1  "UF4_MaintenanceStartSignal"
  Bus Selector4/1 -> UF4_Maintenance State/1(maint_cmd)  "<UF_MaintCmd_4>"
  UF4_BeginStartup/1 -> Bus Selector2/1  "UF4_BeginStartup"
  Bus Selector2/1 -> UF4_Maintenance State/4(startup_cmd)  "<UF_StartupCmd_4>"

== system Ultrafiltration/UF Maintenance Coordinator/arhive/UF_Operation State_5 ==
  UF5_MaintenanceStartSignal : Inport
  UF5_BeginStandby : Inport  Port=2
  UF5_BeginStartup : Inport  Port=3
  Bus Creator : BusCreator  Inputs=2
  Bus Selector : BusSelector  OutputSignals=UF_ShutdownCmd_5
  Bus Selector2 : BusSelector  OutputSignals=UF_StartupCmd_5
  Bus Selector5 : BusSelector  OutputSignals=UF_MaintCmd_5
  Delay Reset Signal : Memory
  Delay Startup : Memory
  UF5_Maintenance State : Stateflow chart  TreatAsAtomicUnit=on
  tag scope: UF5_MaintenanceRequest=global, UF5_MaintenanceState=global, UF5_OperatingState=global, UF5_StartupRequest=global
  wires:
  UF5_Maintenance State/1(unit_in_maint_queue) -> [UF5_MaintenanceRequest]  "UF5_MaintenanceRequestQueue"
  Bus Creator/1 -> [UF5_MaintenanceState]
  Delay Startup/1 -> [UF5_OperatingState], Bus Creator/1  "UF5_OperationsState"
  UF5_Maintenance State/4(maintenance_completion_indicator) -> Delay Reset Signal/1  "UF5_MaintenanceCompletionSignal"
  [UF5_Maintenance_Request] -> UF5_Maintenance State/2(maint_req)
  Delay Reset Signal/1 -> Bus Creator/2  "UF5_MaintenanceCompletionSignal"
  UF5_Maintenance State/3(unit_in_operation) -> Delay Startup/1  "UF5_OperationsState"
  UF5_Maintenance State/2(unit_in_startup_queue) -> [UF5_StartupRequest]  "UF5_StartupRequestQueue"
  UF5_BeginStandby/1 -> Bus Selector/1  "UF5_BeginStandby"
  Bus Selector/1 -> UF5_Maintenance State/3(standby_cmd)  "<UF_ShutdownCmd_5>"
  UF5_MaintenanceStartSignal/1 -> Bus Selector5/1  "UF5_MaintenanceStartSignal"
  Bus Selector5/1 -> UF5_Maintenance State/1(maint_cmd)  "<UF_MaintCmd_5>"
  UF5_BeginStartup/1 -> Bus Selector2/1  "UF5_BeginStartup"
  Bus Selector2/1 -> UF5_Maintenance State/4(startup_cmd)  "<UF_StartupCmd_5>"

== system Ultrafiltration/UF Maintenance Coordinator/arhive/UF_Operation State_6 ==
  UF6_MaintenanceStartSignal : Inport
  UF6_BeginStandby : Inport  Port=2
  UF6_BeginStartup : Inport  Port=3
  Bus Creator : BusCreator  Inputs=2
  Bus Selector : BusSelector  OutputSignals=UF_ShutdownCmd_6
  Bus Selector2 : BusSelector  OutputSignals=UF_StartupCmd_6
  Bus Selector6 : BusSelector  OutputSignals=UF_MaintCmd_6
  Delay Reset Signal : Memory
  Delay Startup : Memory
  UF6_Maintenance State : Stateflow chart  TreatAsAtomicUnit=on
  tag scope: UF6_MaintenanceRequest=global, UF6_MaintenanceState=global, UF6_OperatingState=global, UF6_StartupRequest=global
  wires:
  UF6_Maintenance State/1(unit_in_maint_queue) -> [UF6_MaintenanceRequest]  "UF6_MaintenanceRequestQueue"
  Bus Creator/1 -> [UF6_MaintenanceState]
  Delay Startup/1 -> [UF6_OperatingState], Bus Creator/1  "UF6_OperationsState"
  UF6_Maintenance State/4(maintenance_completion_indicator) -> Delay Reset Signal/1  "UF6_MaintenanceCompletionSignal"
  [UF6_Maintenance_Request] -> UF6_Maintenance State/2(maint_req)
  Delay Reset Signal/1 -> Bus Creator/2  "UF6_MaintenanceCompletionSignal"
  UF6_Maintenance State/3(unit_in_operation) -> Delay Startup/1  "UF6_OperationsState"
  UF6_Maintenance State/2(unit_in_startup_queue) -> [UF6_StartupRequest]  "UF6_StartupRequestQueue"
  UF6_BeginStandby/1 -> Bus Selector/1  "UF6_BeginStandby"
  Bus Selector/1 -> UF6_Maintenance State/3(standby_cmd)  "<UF_ShutdownCmd_6>"
  UF6_MaintenanceStartSignal/1 -> Bus Selector6/1  "UF6_MaintenanceStartSignal"
  Bus Selector6/1 -> UF6_Maintenance State/1(maint_cmd)  "<UF_MaintCmd_6>"
  UF6_BeginStartup/1 -> Bus Selector2/1  "UF6_BeginStartup"
  Bus Selector2/1 -> UF6_Maintenance State/4(startup_cmd)  "<UF_StartupCmd_6>"
